simulink model "DreiTankSim_Visual"  (R2021a)
settings: Solver=ode5  StartTime=0.0  StopTime=inf  RelTol=1e-3
model workspace (MAT data in the model file):
  A1 = 20
  A2 = 20
  A3 = 20
  Kt = 1
  Kv = 8.75529661017
  Kvgekop = 6.21621117085
  k1 = 1.5
  k2 = 1.5
  k3 = 1.5
  k4 = 5
  k5 = 5
  k6 = 5
libraries: pid_lib x3, sldrtlib x3
(part 2 of 2)

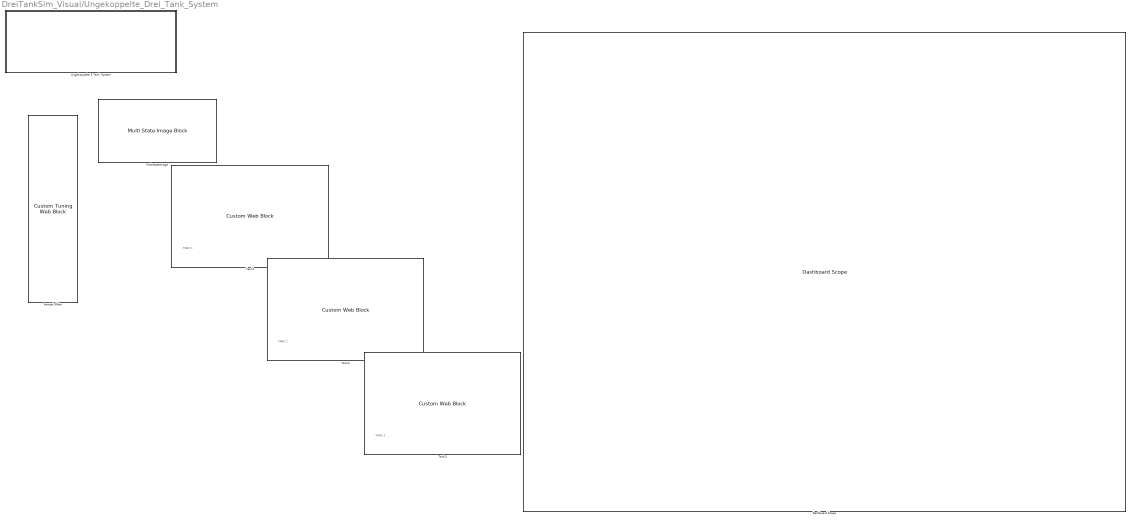
== system DreiTankSim_Visual/Ungekoppelte_Drei_Tank_System ==
  note: TANK 1
  note: TANK 2
  note: TANK 3
  Dashboard Scope : DashboardScope  Ymin=0  Ymax=300  LegendPosition=Right  ScaleAtStop=off  UpdateMode=Scroll
  MultiStateImage : MultiStateImageBlock  LabelPosition=Hide  ScaleMode=Fill
  Tank1 : CustomWebBlock  LabelPosition=Hide  ShowInitialText=on  Configuration="{\"components\":[{\"name\":\"LinearScaleComponent\",\"settings\":{\"bounds\":{\"max\":200,\"min\":0,\"tickInterval\":\"auto\"},\"internalTickHeightScaleFactor\":0.5,\"labelColor\":[0,255,0],\"labelFont\":{\"font\":\"Arial\",\"fontSize\":12},\"labelTransparency\":0.5,\"needleImage\":{\"size\":[21,75],\"src\":\"data:image\\/svg+xml;base64,PHN2ZyB4bWxucz0iaHR0cDovL3d3dy53My5vcmcvMjAwMC9zdmciIHhtbG5zOnhsaW5rPSJodHRwOi8vd3d3LnczLm9yZy8xOTk5L3hsaW5rIiB2aWV3Qm94PSIwIDAgMjEgNzUiPjxkZWZzPjxzdHlsZT4uY2xzLTF7ZmlsbDpub25lO30uY2xzLTJ7aXNvbGF0aW9uOmlzb2xhdGU7fS5jbHMtM3tjbGlwLXBhdGg6dXJsKCNjbGlwLXBhdGgpO30uY2xzLTR7b3BhY2l0eTowLjM7bWl4LWJsZW5kLW1vZGU6bXVsdGlwbHk7fS5jbHMtNXtmaWxsOiNlYjI2Mjk7fTwvc3R5bGU+PGNsaXBQYXRoIGlkPSJjbGlwLXBhdGgiIHRyYW5zZm9y ...(+1928 chars)\",\"srcOrientation\":\"horizontal\"},\"needleOffset\":[-0.01094391244870041,0],\"needleSize\":{\"height\":0.06,\"width\":0.48},\"position\":[0.010036879697493114,0.05628619691119691,0.4390685328185328,0.761262312683815],\"scaleColors\":[],\"scaleColorsSize\":0.2,\"showLabels\":1,\"showMinorTicks\":0,\"showSpanLine\":1,\"showTicks\":1,\"tickColor\":[204,204,204],\"tickTransparency\":0.5,\"valueBarColor\":[127,205,255],\"valueBarOffset\":0,\"valueBarSize\":0.95,\"valueBarTransparency\":1}},{\"name\":\"BackgroundImageComponent\",\"settings\":{\"image\":{\"size\":[267,174],\"src\":\"data:image\\/png;base64,iVBORw0KGgoAAAANSUhEUgAAAQsAAACuCAYAAAAh8yi7AAAACXBIWXMAABJ0AAASdAHeZh94AAAGS0lEQVR4Xu3d4W4TOxAGUEC8\\/yO3EESlUqD5HI83u+ODdH8gvF7PmeHLNqW5X774RYAAAQIECBAgQIAAAQIECBAgQIAAAQIECBAgQIAAAQIECBAgQIAAAQIECBAgQIAAAQInFPg6eaaXd9ff9nr9+d+3yT1d\\/jyBWz\\/fz4R+Pq8Xp7vz94ITzQZOwRFsQYDAagFPAauF7U+giUB1WHjKuPZg6N+1+7f09LNhYbiWtufpm+vv01twngPMhsV5KnESAgSWCgiLpbyX3\\/z23RC\\/CPwSEBYGgQCBSKA6LLwSRewWEbieQHVYXE\\/A ...(+1892 chars)\",\"srcOrientation\":\"vertical\"},\"position\":[0,0,1,1],\"scaleMode\":\"0\"}},{\"name\":\"ForegroundImageComponent\",\"settings\":{\"image\":{\"size\":[0,0],\"src\":\"default\",\"srcOrientation\":[]},\"isForeground\":1,\"position\":[0,0,1,1],\"scaleMode\":\"0\"}}],\"settings\":{\"BindingType\":\"signal\",\"backgroundColor\":[255,255,255,\"1\"],\"backgroundOffset\":0,\"backgroundOpacity\":0,\"fixedAspectRatio\":\"on\",\"orientation\":\"vertical\",\"showBackgroundColor\":false,\"value\":0},\"type\":\"LinearGauge\"}"
  Tank2 : CustomWebBlock  LabelPosition=Hide  ShowInitialText=on  Configuration="{\"components\":[{\"name\":\"LinearScaleComponent\",\"settings\":{\"bounds\":{\"max\":200,\"min\":0,\"tickInterval\":\"auto\"},\"internalTickHeightScaleFactor\":0.5,\"labelColor\":[0,255,0],\"labelFont\":{\"font\":\"Arial\",\"fontSize\":12},\"labelTransparency\":0.5,\"needleImage\":{\"size\":[21,75],\"src\":\"data:image\\/svg+xml;base64,PHN2ZyB4bWxucz0iaHR0cDovL3d3dy53My5vcmcvMjAwMC9zdmciIHhtbG5zOnhsaW5rPSJodHRwOi8vd3d3LnczLm9yZy8xOTk5L3hsaW5rIiB2aWV3Qm94PSIwIDAgMjEgNzUiPjxkZWZzPjxzdHlsZT4uY2xzLTF7ZmlsbDpub25lO30uY2xzLTJ7aXNvbGF0aW9uOmlzb2xhdGU7fS5jbHMtM3tjbGlwLXBhdGg6dXJsKCNjbGlwLXBhdGgpO30uY2xzLTR7b3BhY2l0eTowLjM7bWl4LWJsZW5kLW1vZGU6bXVsdGlwbHk7fS5jbHMtNXtmaWxsOiNlYjI2Mjk7fTwvc3R5bGU+PGNsaXBQYXRoIGlkPSJjbGlwLXBhdGgiIHRyYW5zZm9y ...(+1928 chars)\",\"srcOrientation\":\"horizontal\"},\"needleOffset\":[-0.01094391244870041,0],\"needleSize\":{\"height\":0.06,\"width\":0.48},\"position\":[0.010036879697493114,0.05628619691119691,0.4371380308880309,0.7582745903552589],\"scaleColors\":[],\"scaleColorsSize\":0.2,\"showLabels\":1,\"showMinorTicks\":0,\"showSpanLine\":1,\"showTicks\":1,\"tickColor\":[204,204,204],\"tickTransparency\":0.5,\"valueBarColor\":[127,205,255],\"valueBarOffset\":0,\"valueBarSize\":0.95,\"valueBarTransparency\":1}},{\"name\":\"BackgroundImageComponent\",\"settings\":{\"image\":{\"size\":[267,174],\"src\":\"data:image\\/png;base64,iVBORw0KGgoAAAANSUhEUgAAAQsAAACuCAYAAAAh8yi7AAAACXBIWXMAABJ0AAASdAHeZh94AAAGS0lEQVR4Xu3d4W4TOxAGUEC8\\/yO3EESlUqD5HI83u+ODdH8gvF7PmeHLNqW5X774RYAAAQIECBAgQIAAAQIECBAgQIAAAQIECBAgQIAAAQIECBAgQIAAAQIECBAgQIAAAQInFPg6eaaXd9ff9nr9+d+3yT1d\\/jyBWz\\/fz4R+Pq8Xp7vz94ITzQZOwRFsQYDAagFPAauF7U+giUB1WHjKuPZg6N+1+7f09LNhYbiWtufpm+vv01twngPMhsV5KnESAgSWCgiLpbyX3\\/z23RC\\/CPwSEBYGgQCBSKA6LLwSRewWEbieQHVYXE\\/A ...(+1892 chars)\",\"srcOrientation\":\"vertical\"},\"position\":[0,0,1,1],\"scaleMode\":\"0\"}},{\"name\":\"ForegroundImageComponent\",\"settings\":{\"image\":{\"size\":[0,0],\"src\":\"default\",\"srcOrientation\":[]},\"isForeground\":1,\"position\":[0,0,1,1],\"scaleMode\":\"0\"}}],\"settings\":{\"BindingType\":\"signal\",\"backgroundColor\":[255,255,255,\"1\"],\"backgroundOffset\":0,\"backgroundOpacity\":0,\"fixedAspectRatio\":\"on\",\"orientation\":\"vertical\",\"showBackgroundColor\":false,\"value\":147.88},\"type\":\"LinearGauge\"}"
  Tank3 : CustomWebBlock  LabelPosition=Hide  ShowInitialText=on  Configuration="{\"components\":[{\"name\":\"LinearScaleComponent\",\"settings\":{\"bounds\":{\"max\":200,\"min\":0,\"tickInterval\":\"auto\"},\"internalTickHeightScaleFactor\":0.5,\"labelColor\":[0,255,0],\"labelFont\":{\"font\":\"Arial\",\"fontSize\":12},\"labelTransparency\":0.5,\"needleImage\":{\"size\":[21,75],\"src\":\"data:image\\/svg+xml;base64,PHN2ZyB4bWxucz0iaHR0cDovL3d3dy53My5vcmcvMjAwMC9zdmciIHhtbG5zOnhsaW5rPSJodHRwOi8vd3d3LnczLm9yZy8xOTk5L3hsaW5rIiB2aWV3Qm94PSIwIDAgMjEgNzUiPjxkZWZzPjxzdHlsZT4uY2xzLTF7ZmlsbDpub25lO30uY2xzLTJ7aXNvbGF0aW9uOmlzb2xhdGU7fS5jbHMtM3tjbGlwLXBhdGg6dXJsKCNjbGlwLXBhdGgpO30uY2xzLTR7b3BhY2l0eTowLjM7bWl4LWJsZW5kLW1vZGU6bXVsdGlwbHk7fS5jbHMtNXtmaWxsOiNlYjI2Mjk7fTwvc3R5bGU+PGNsaXBQYXRoIGlkPSJjbGlwLXBhdGgiIHRyYW5zZm9y ...(+1928 chars)\",\"srcOrientation\":\"horizontal\"},\"needleOffset\":[-0.01094391244870041,0],\"needleSize\":{\"height\":0.06,\"width\":0.48},\"position\":[0.017523364485981307,0.057669082125603864,0.4331597222222222,0.7507593457943925],\"scaleColors\":[],\"scaleColorsSize\":0.2,\"showLabels\":1,\"showMinorTicks\":0,\"showSpanLine\":1,\"showTicks\":1,\"tickColor\":[204,204,204],\"tickTransparency\":0.5,\"valueBarColor\":[127,205,255],\"valueBarOffset\":0,\"valueBarSize\":0.95,\"valueBarTransparency\":1}},{\"name\":\"BackgroundImageComponent\",\"settings\":{\"image\":{\"size\":[267,174],\"src\":\"data:image\\/png;base64,iVBORw0KGgoAAAANSUhEUgAAAQsAAACuCAYAAAAh8yi7AAAACXBIWXMAABJ0AAASdAHeZh94AAAGS0lEQVR4Xu3d4W4TOxAGUEC8\\/yO3EESlUqD5HI83u+ODdH8gvF7PmeHLNqW5X774RYAAAQIECBAgQIAAAQIECBAgQIAAAQIECBAgQIAAAQIECBAgQIAAAQIECBAgQIAAAQInFPg6eaaXd9ff9nr9+d+3yT1d\\/jyBWz\\/fz4R+Pq8Xp7vz94ITzQZOwRFsQYDAagFPAauF7U+giUB1WHjKuPZg6N+1+7f09LNhYbiWtufpm+vv01twngPMhsV5KnESAgSWCgiLpbyX3\\/z23RC\\/CPwSEBYGgQCBSKA6LLwSRewWEbieQHVYXE\\/A ...(+1892 chars)\",\"srcOrientation\":\"vertical\"},\"position\":[0,0,1,1],\"scaleMode\":\"0\"}},{\"name\":\"ForegroundImageComponent\",\"settings\":{\"image\":{\"size\":[0,0],\"src\":\"default\",\"srcOrientation\":[]},\"isForeground\":1,\"position\":[0,0,1,1],\"scaleMode\":\"0\"}}],\"settings\":{\"BindingType\":\"signal\",\"backgroundColor\":[255,255,255,\"1\"],\"backgroundOffset\":0,\"backgroundOpacity\":0,\"fixedAspectRatio\":\"on\",\"orientation\":\"vertical\",\"showBackgroundColor\":false,\"value\":0},\"type\":\"LinearGauge\"}"
  "Ungekoppelte 3 Tank System " : Subsystem
      mask Display: image('C:\Users\Oğulcan\OneDrive\Masaüstü\GörOgiProjekt\MatlabGUİ\GuiTemiz\Taulogo.png'); % Use "Edit Image" on toolstrip to change.
  Vertical Slider : CustomTuningWebBlock  LabelPosition=Hide  ShowInitialText=on  Configuration="{\"components\":[{\"name\":\"LinearScaleComponent\",\"settings\":{\"bounds\":{\"max\":20,\"min\":0,\"tickInterval\":1},\"internalTickHeightScaleFactor\":1,\"labelColor\":[255,255,0],\"labelFont\":{\"font\":\"Arial\",\"fontSize\":12},\"labelOffset\":0.05,\"labelTransparency\":1,\"needleImage\":{\"size\":[842,596],\"src\":\"data:image\\/svg+xml;base64,PD94bWwgdmVyc2lvbj0iMS4wIiBlbmNvZGluZz0idXRmLTgiPz4NCjwhLS0gR2VuZXJhdG9yOiBBZG9iZSBJbGx1c3RyYXRvciAyNS4wLjAsIFNWRyBFeHBvcnQgUGx1Zy1JbiAuIFNWRyBWZXJzaW9uOiA2LjAwIEJ1aWxkIDApICAtLT4NCjxzdmcgdmVyc2lvbj0iMS4xIg0KCSBpZD0ic3ZnOCIgeG1sbnM6Y2M9Imh0dHA6Ly9jcmVhdGl2ZWNvbW1vbnMub3JnL25zIyIgeG1sbnM6ZGM9Imh0dHA6Ly9wdXJsLm9yZy9kYy9lbGVtZW50cy8xLjEvIiB4bWxuczppbmtzY2FwZT0iaHR0cDovL3d3dy5pbmtzY2FwZS5vcmcvbmFtZXNw ...(+2376 chars)\",\"srcOrientation\":\"vertical\"},\"needleOffset\":[0.02,-0.8],\"needleSize\":{\"height\":0.07532387955182072,\"width\":0.43386243386243384},\"position\":[0.027412280701754384,0.2830188679245283,0.5832841981132075,0.9524201127819549],\"scaleColors\":[],\"scaleColorsSize\":0.2,\"showLabels\":1,\"showMinorTicks\":0,\"showSpanLine\":1,\"showTicks\":1,\"tickColor\":[234,234,234],\"tickTransparency\":1,\"valueBarColor\":[0,255,255],\"valueBarOffset\":-0.3,\"valueBarSize\":0.15,\"valueBarTransparency\":1}},{\"name\":\"BackgroundImageComponent\",\"settings\":{\"image\":{\"size\":[101,380],\"src\":\"data:image\\/svg+xml;base64,PD94bWwgdmVyc2lvbj0iMS4wIiBlbmNvZGluZz0iVVRGLTgiIHN0YW5kYWxvbmU9Im5vIj8+CjxzdmcKICAgeG1sbnM6ZGM9Imh0dHA6Ly9wdXJsLm9yZy9kYy9lbGVtZW50cy8xLjEvIgogICB4bWxuczpjYz0iaHR0cDovL2NyZWF0aXZlY29tbW9ucy5vcmcvbnMjIgogICB4bWxuczpyZGY9Imh0dHA6Ly93d3cudzMub3JnLzE5OTkvMDIvMjItcmRmLXN5bnRheC1ucyMiCiAgIHhtbG5zOnN2Zz0iaHR0cDovL3d3dy53My5vcmcvMjAwMC9zdmciCiAgIHhtbG5zPSJodHRwOi8vd3d3LnczLm9yZy8yMDAwL3N2ZyIKICAgeG1sbnM6 ...(+3116 chars)\",\"srcOrientation\":\"vertical\"},\"position\":[0,0,1,1],\"scaleMode\":\"0\"}},{\"name\":\"ForegroundImageComponent\",\"settings\":{\"image\":{\"size\":[0,0],\"src\":\"default\",\"srcOrientation\":null},\"isForeground\":1,\"position\":[0,0,1,1],\"scaleMode\":\"0\"}}],\"settings\":{\"BindingType\":\"param\",\"aspectRatio\":0.2651006711409396,\"backgroundColor\":[0,0,0,\"1\"],\"backgroundOffset\":0,\"backgroundOpacity\":1,\"fixedAspectRatio\":\"on\",\"orientation\":\"vertical\",\"showBackgroundColor\":false,\"value\":0},\"type\":\"LinearGauge\"}"

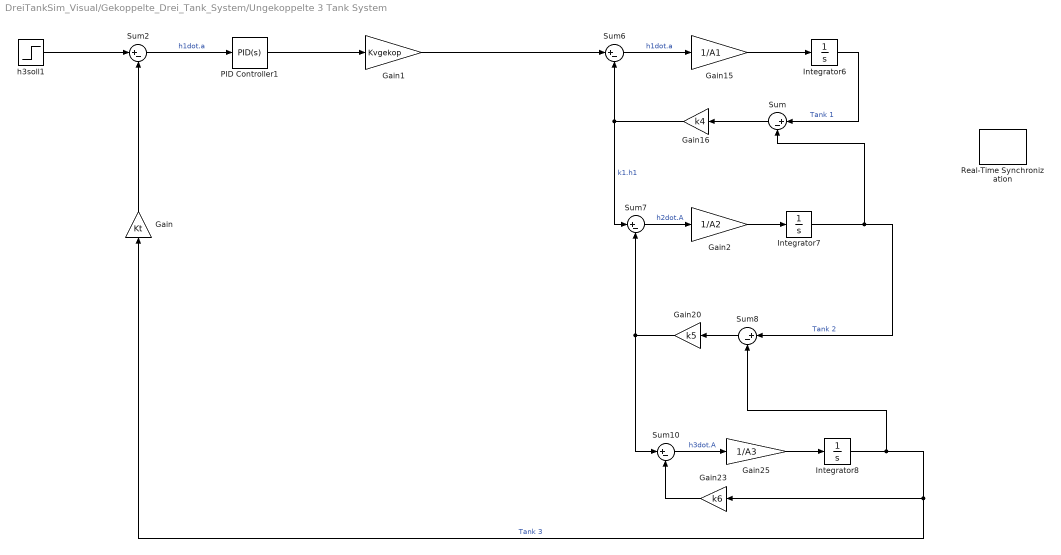
== system DreiTankSim_Visual/Gekoppelte_Drei_Tank_System/Ungekoppelte 3 Tank System  ==
  Gain : Gain  Gain=Kt
  Gain1 : Gain  Gain=Kvgekop
  Gain15 : Gain  Gain=1/A1
  Gain16 : Gain  Gain=k4
  Gain2 : Gain  Gain=1/A2
  Gain20 : Gain  Gain=k5
  Gain23 : Gain  Gain=k6
  Gain25 : Gain  Gain=1/A3
  Integrator6 : Integrator
  Integrator7 : Integrator
  Integrator8 : Integrator
  PID Controller1 : pid_lib/PID Controller  Controller=PID  Form=Ideal  TimeDomain=Continuous-time  UseExternalTs=off  SampleTime=-1  IntegratorMethod=Forward Euler  FilterMethod=Forward Euler  ControllerParametersSource=internal  P=2  I=0.05  D=0  UseFilter=on  N=100  TunerSelectOption=Transfer Function Based (PID Tuner App)  InitialConditionSource=internal  InitialConditionForIntegrator=0  InitialConditionForFilter=0  DifferentiatorICPrevScaledInput=0  ExternalReset=none  TrackingMode=off  Kt=1  LimitOutput=off  SatLimitsSource=internal  UpperSaturationLimit=inf  LowerSaturationLimit=-inf  LinearizeAsGain=on  AntiWindupMode=none  Kb=1  POutMin=[]  POutMax=[]  IOutMin=[]  IOutMax=[]  DOutMin=[]  DOutMax=[]  NOutMin=[]  NOutMax=[]  SumOutMin=[]  SumOutMax=[]  SaturationOutMin=[]  SaturationOutMax=[]  PParamMin=[]  PParamMax=[]  IParamMin=[]  IParamMax=[]  DParamMin=[]  DParamMax=[]  NParamMin=[]  NParamMax=[]  KbParamMin=[]  KbParamMax=[]  KtParamMin=[]  KtParamMax=[]  KbOutMin=[]  KbOutMax=[]  KtOutMin=[]  KtOutMax=[]  IntegratorOutMin=[]  IntegratorOutMax=[]  FilterOutMin=[]  FilterOutMax=[]  SumI1OutMin=[]  SumI1OutMax=[]  SumI2OutMin=[]  SumI2OutMax=[]  SumI3OutMin=[]  SumI3OutMax=[]  SumI4OutMin=[]  SumI4OutMax=[]  SumDOutMin=[]  SumDOutMax=[]  DifferentiatorOutMin=[]  DifferentiatorOutMax=[]  FilterDiffOutCoefMin=[]  FilterDiffOutCoefMax=[]  ReciprocalOutMin=[]  ReciprocalOutMax=[]  SumDenOutMin=[]  SumDenOutMax=[]  SumNumOutMin=[]  SumNumOutMax=[]  DivideOutMin=[]  DivideOutMax=[]  UdiffTsProdOutMin=[]  UdiffTsProdOutMax=[]  NTsProdOutMin=[]  NTsProdOutMax=[]  UintegralTsProdOutMin=[]  UintegralTsProdOutMax=[]  UngainTsProdOutMin=[]  UngainTsProdOutMax=[]  IntegratorContinuousStateAttributes=''  IntegratorStateMustResolveToSignalObject=off  IntegratorRTWStateStorageClass=Auto  FilterContinuousStateAttributes=''  FilterStateMustResolveToSignalObject=off  FilterRTWStateStorageClass=Auto  ParallelPVariant=Passthrough  IdealPVariant=InternalParameters  IVariant=InternalParameters  DVariant=InternalParameters  IntegratorVariant=Continuous  SatVariant=Disabled  AWVariant=Passthrough  PCopyVariant=Disabled  TRVariant=Disabled  FdbkBlocksVariant=Forward  IdealPFdbkVariant=Disabled  SatFdbkVariant=Disabled  DerivativeFilterVariant=ContFilter  NVariant=InternalParameters  NCopyVariant=Disabled  FilterICVariant=InternalICsFilter  IntegratorICVariant=InternalICs  ExternalResetVariant=Disabled  TRSumVariant=Passthrough  SumFdbkVariant=Disabled  SumVariant=Sum_PID  TsampFilterVariant=InternalTs  TsampNgainVariant=Passthrough  TsampIntegralVariant=Passthrough  ExternalSaturationOutDataTypeStr=Inherit: Same as second input
  Real-Time Synchronization : sldrtlib/Real-Time Synchronization  SampleTime=0.1  MaxMissedTicks=1000  ShowMissedTicks=off  YieldWhenWaiting=off
  Sum{,2,6..8,10} (6 alike) : Sum  Inputs=|+-
  h3soll1 : Step  After=1000  SampleTime=0
  wires:
  Gain/1 -> Sum2/2
  Gain23/1 -> Sum10/2
  Gain20/1 -> Sum10/1, Sum7/2
  Sum7/1 -> Gain2/1  "h2dot.A"
  Integrator6/1 -> Sum/1  "Tank 1"
  Sum/1 -> Gain16/1
  Gain16/1 -> Sum6/2, Sum7/1  "k1.h1"
  Gain15/1 -> Integrator6/1
  Sum8/1 -> Gain20/1
  Integrator7/1 -> Sum/2, Sum8/1  "Tank 2"
  Gain25/1 -> Integrator8/1
  Sum10/1 -> Gain25/1  "h3dot.A"
  Gain2/1 -> Integrator7/1
  Integrator8/1 -> Sum8/2, Gain/1, Gain23/1  "Tank 3"
  Sum6/1 -> Gain15/1  "h1dot.a"
  Gain1/1 -> Sum6/1
  PID Controller1/1 -> Gain1/1
  h3soll1/1 -> Sum2/1
  Sum2/1 -> PID Controller1/1  "h1dot.a"

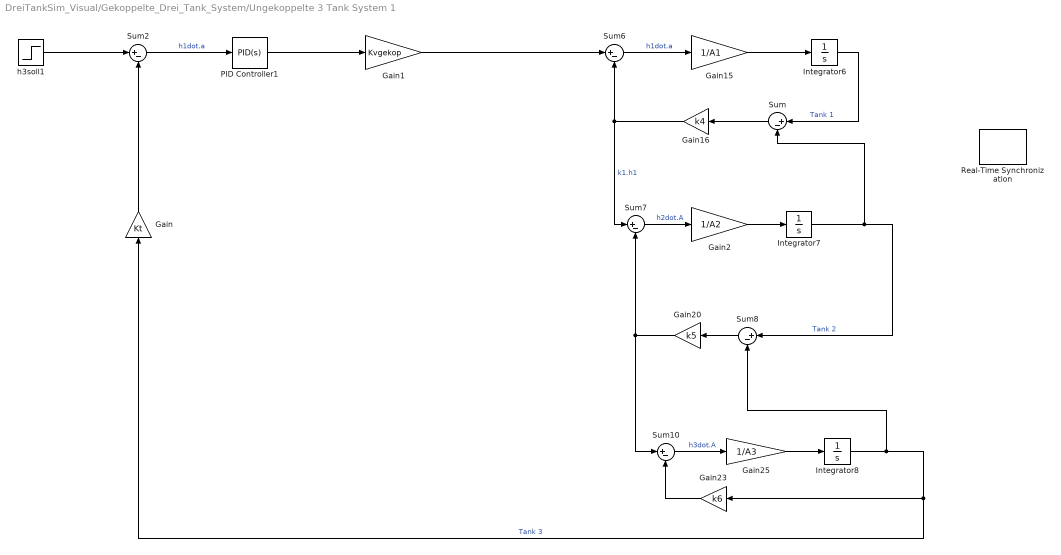
== system DreiTankSim_Visual/Gekoppelte_Drei_Tank_System/Ungekoppelte 3 Tank System 1 ==
  Gain : Gain  Gain=Kt
  Gain1 : Gain  Gain=Kvgekop
  Gain15 : Gain  Gain=1/A1
  Gain16 : Gain  Gain=k4
  Gain2 : Gain  Gain=1/A2
  Gain20 : Gain  Gain=k5
  Gain23 : Gain  Gain=k6
  Gain25 : Gain  Gain=1/A3
  Integrator6 : Integrator
  Integrator7 : Integrator
  Integrator8 : Integrator
  PID Controller1 : pid_lib/PID Controller  Controller=PID  Form=Ideal  TimeDomain=Continuous-time  UseExternalTs=off  SampleTime=-1  IntegratorMethod=Forward Euler  FilterMethod=Forward Euler  ControllerParametersSource=internal  P=2  I=0.05  D=0  UseFilter=on  N=100  TunerSelectOption=Transfer Function Based (PID Tuner App)  InitialConditionSource=internal  InitialConditionForIntegrator=0  InitialConditionForFilter=0  DifferentiatorICPrevScaledInput=0  ExternalReset=none  TrackingMode=off  Kt=1  LimitOutput=off  SatLimitsSource=internal  UpperSaturationLimit=inf  LowerSaturationLimit=-inf  LinearizeAsGain=on  AntiWindupMode=none  Kb=1  POutMin=[]  POutMax=[]  IOutMin=[]  IOutMax=[]  DOutMin=[]  DOutMax=[]  NOutMin=[]  NOutMax=[]  SumOutMin=[]  SumOutMax=[]  SaturationOutMin=[]  SaturationOutMax=[]  PParamMin=[]  PParamMax=[]  IParamMin=[]  IParamMax=[]  DParamMin=[]  DParamMax=[]  NParamMin=[]  NParamMax=[]  KbParamMin=[]  KbParamMax=[]  KtParamMin=[]  KtParamMax=[]  KbOutMin=[]  KbOutMax=[]  KtOutMin=[]  KtOutMax=[]  IntegratorOutMin=[]  IntegratorOutMax=[]  FilterOutMin=[]  FilterOutMax=[]  SumI1OutMin=[]  SumI1OutMax=[]  SumI2OutMin=[]  SumI2OutMax=[]  SumI3OutMin=[]  SumI3OutMax=[]  SumI4OutMin=[]  SumI4OutMax=[]  SumDOutMin=[]  SumDOutMax=[]  DifferentiatorOutMin=[]  DifferentiatorOutMax=[]  FilterDiffOutCoefMin=[]  FilterDiffOutCoefMax=[]  ReciprocalOutMin=[]  ReciprocalOutMax=[]  SumDenOutMin=[]  SumDenOutMax=[]  SumNumOutMin=[]  SumNumOutMax=[]  DivideOutMin=[]  DivideOutMax=[]  UdiffTsProdOutMin=[]  UdiffTsProdOutMax=[]  NTsProdOutMin=[]  NTsProdOutMax=[]  UintegralTsProdOutMin=[]  UintegralTsProdOutMax=[]  UngainTsProdOutMin=[]  UngainTsProdOutMax=[]  IntegratorContinuousStateAttributes=''  IntegratorStateMustResolveToSignalObject=off  IntegratorRTWStateStorageClass=Auto  FilterContinuousStateAttributes=''  FilterStateMustResolveToSignalObject=off  FilterRTWStateStorageClass=Auto  ParallelPVariant=Passthrough  IdealPVariant=InternalParameters  IVariant=InternalParameters  DVariant=InternalParameters  IntegratorVariant=Continuous  SatVariant=Disabled  AWVariant=Passthrough  PCopyVariant=Disabled  TRVariant=Disabled  FdbkBlocksVariant=Forward  IdealPFdbkVariant=Disabled  SatFdbkVariant=Disabled  DerivativeFilterVariant=ContFilter  NVariant=InternalParameters  NCopyVariant=Disabled  FilterICVariant=InternalICsFilter  IntegratorICVariant=InternalICs  ExternalResetVariant=Disabled  TRSumVariant=Passthrough  SumFdbkVariant=Disabled  SumVariant=Sum_PID  TsampFilterVariant=InternalTs  TsampNgainVariant=Passthrough  TsampIntegralVariant=Passthrough  ExternalSaturationOutDataTypeStr=Inherit: Same as second input
  Real-Time Synchronization : sldrtlib/Real-Time Synchronization  SampleTime=0.1  MaxMissedTicks=1000  ShowMissedTicks=off  YieldWhenWaiting=off
  Sum{,2,6..8,10} (6 alike) : Sum  Inputs=|+-
  h3soll1 : Step  After=1000  SampleTime=0
  wires:
  Sum2/1 -> PID Controller1/1  "h1dot.a"
  h3soll1/1 -> Sum2/1
  PID Controller1/1 -> Gain1/1
  Gain1/1 -> Sum6/1
  Sum6/1 -> Gain15/1  "h1dot.a"
  Integrator8/1 -> Gain23/1, Gain/1, Sum8/2  "Tank 3"
  Gain2/1 -> Integrator7/1
  Sum10/1 -> Gain25/1  "h3dot.A"
  Gain25/1 -> Integrator8/1
  Integrator7/1 -> Sum8/1, Sum/2  "Tank 2"
  Sum8/1 -> Gain20/1
  Gain15/1 -> Integrator6/1
  Gain16/1 -> Sum7/1, Sum6/2  "k1.h1"
  Sum/1 -> Gain16/1
  Integrator6/1 -> Sum/1  "Tank 1"
  Sum7/1 -> Gain2/1  "h2dot.A"
  Gain20/1 -> Sum7/2, Sum10/1
  Gain23/1 -> Sum10/2
  Gain/1 -> Sum2/2

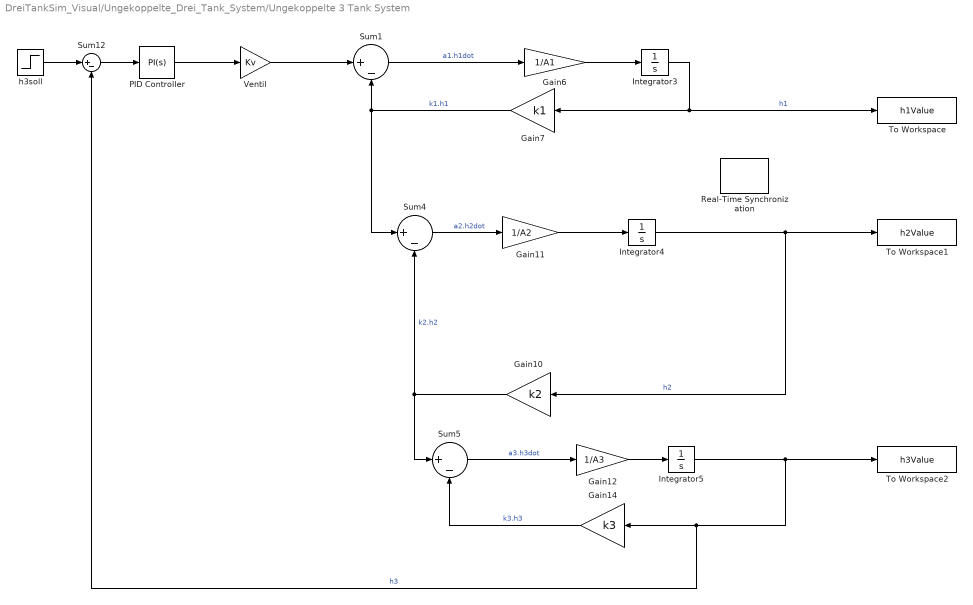
== system DreiTankSim_Visual/Ungekoppelte_Drei_Tank_System/Ungekoppelte 3 Tank System  ==
  Gain10 : Gain  Gain=k2
  Gain11 : Gain  Gain=1/A2
  Gain12 : Gain  Gain=1/A3
  Gain14 : Gain  Gain=k3
  Gain6 : Gain  Gain=1/A1
  Gain7 : Gain  Gain=k1
  Integrator3 : Integrator
  Integrator4 : Integrator
  Integrator5 : Integrator
  PID Controller : pid_lib/PID Controller  Controller=PI  Form=Ideal  TimeDomain=Continuous-time  UseExternalTs=off  SampleTime=-1  IntegratorMethod=Forward Euler  FilterMethod=Forward Euler  ControllerParametersSource=internal  P=0.1  I=0.05  D=0  UseFilter=on  N=100  TunerSelectOption=Transfer Function Based (PID Tuner App)  InitialConditionSource=internal  InitialConditionForIntegrator=0  InitialConditionForFilter=0  DifferentiatorICPrevScaledInput=0  ExternalReset=none  TrackingMode=off  Kt=1  LimitOutput=off  SatLimitsSource=internal  UpperSaturationLimit=inf  LowerSaturationLimit=-inf  LinearizeAsGain=on  AntiWindupMode=none  Kb=1  POutMin=[]  POutMax=[]  IOutMin=[]  IOutMax=[]  DOutMin=[]  DOutMax=[]  NOutMin=[]  NOutMax=[]  SumOutMin=[]  SumOutMax=[]  SaturationOutMin=[]  SaturationOutMax=[]  PParamMin=[]  PParamMax=[]  IParamMin=[]  IParamMax=[]  DParamMin=[]  DParamMax=[]  NParamMin=[]  NParamMax=[]  KbParamMin=[]  KbParamMax=[]  KtParamMin=[]  KtParamMax=[]  KbOutMin=[]  KbOutMax=[]  KtOutMin=[]  KtOutMax=[]  IntegratorOutMin=[]  IntegratorOutMax=[]  FilterOutMin=[]  FilterOutMax=[]  SumI1OutMin=[]  SumI1OutMax=[]  SumI2OutMin=[]  SumI2OutMax=[]  SumI3OutMin=[]  SumI3OutMax=[]  SumI4OutMin=[]  SumI4OutMax=[]  SumDOutMin=[]  SumDOutMax=[]  DifferentiatorOutMin=[]  DifferentiatorOutMax=[]  FilterDiffOutCoefMin=[]  FilterDiffOutCoefMax=[]  ReciprocalOutMin=[]  ReciprocalOutMax=[]  SumDenOutMin=[]  SumDenOutMax=[]  SumNumOutMin=[]  SumNumOutMax=[]  DivideOutMin=[]  DivideOutMax=[]  UdiffTsProdOutMin=[]  UdiffTsProdOutMax=[]  NTsProdOutMin=[]  NTsProdOutMax=[]  UintegralTsProdOutMin=[]  UintegralTsProdOutMax=[]  UngainTsProdOutMin=[]  UngainTsProdOutMax=[]  IntegratorContinuousStateAttributes=''  IntegratorStateMustResolveToSignalObject=off  IntegratorRTWStateStorageClass=Auto  FilterContinuousStateAttributes=''  FilterStateMustResolveToSignalObject=off  FilterRTWStateStorageClass=Auto  ParallelPVariant=Passthrough  IdealPVariant=InternalParameters  IVariant=InternalParameters  DVariant=Disabled  IntegratorVariant=Continuous  SatVariant=Disabled  AWVariant=Passthrough  PCopyVariant=Disabled  TRVariant=Disabled  FdbkBlocksVariant=Forward  IdealPFdbkVariant=Disabled  SatFdbkVariant=Disabled  DerivativeFilterVariant=Disabled  NVariant=Disabled  NCopyVariant=Disabled_SignalSpec  FilterICVariant=Disabled  IntegratorICVariant=InternalICs  ExternalResetVariant=Disabled  TRSumVariant=Passthrough  SumFdbkVariant=Disabled  SumVariant=Sum_PI  TsampFilterVariant=InternalTs  TsampNgainVariant=Passthrough  TsampIntegralVariant=Passthrough  ExternalSaturationOutDataTypeStr=Inherit: Same as second input
  Real-Time Synchronization : sldrtlib/Real-Time Synchronization  SampleTime=0.1  MaxMissedTicks=1000  ShowMissedTicks=off  YieldWhenWaiting=off
  Sum{1,4..5,12} (4 alike) : Sum  Inputs=|+-
  To Workspace : ToWorkspace  VariableName=h1Value  SaveFormat=Timeseries  SampleTime=-1
  To Workspace1 : ToWorkspace  VariableName=h2Value  SaveFormat=Timeseries  SampleTime=-1
  To Workspace2 : ToWorkspace  VariableName=h3Value  SaveFormat=Timeseries  SampleTime=-1
  Ventil : Gain  Gain=Kv
  h3soll : Step  After=100  SampleTime=0
  wires:
  Gain7/1 -> Sum1/2, Sum4/1  "k1.h1"
  Gain14/1 -> Sum5/2  "k3.h3"
  Integrator5/1 -> Sum12/2, Gain14/1, To Workspace2/1  "h3"
  Sum1/1 -> Gain6/1  "a1.h1dot"
  Integrator4/1 -> To Workspace1/1, Gain10/1  "h2"
  PID Controller/1 -> Ventil/1
  Gain11/1 -> Integrator4/1
  Gain6/1 -> Integrator3/1
  Sum5/1 -> Gain12/1  "a3.h3dot"
  h3soll/1 -> Sum12/1
  Gain10/1 -> Sum4/2, Sum5/1  "k2.h2"
  Sum12/1 -> PID Controller/1
  Ventil/1 -> Sum1/1
  Gain12/1 -> Integrator5/1
  Sum4/1 -> Gain11/1  "a2.h2dot"
  Integrator3/1 -> Gain7/1, To Workspace/1  "h1"
